simulink model "ASM_Traffic_V2X_Complete_Model_2"  (R2019a)
settings: Solver=ode1  StartTime=SIM.tstart.v  StopTime=Inf  FixedStep=SIM.StepSize.v  RelTol=1e-3
PostLoadFcn:
  | if any(exist('dsrtsu_mdlpostloadfcn', 'file') ~= 0), dsrtsu_mdlpostloadfcn('Execute', bdroot); end
  | try, asm_mdl_postloadfcn(bdroot, 'UpdateModel', 2200); catch, disp(lasterr); end,
undefined symbols (not defined in the file): _SensorPnts_1, _SensorPnts_13, _SensorPnts_17, _SensorPnts_21, _SensorPnts_25, _SensorPnts_29, _SensorPnts_33, _SensorPnts_37, _SensorPnts_41, _SensorPnts_45, _SensorPnts_49, _SensorPnts_5, _SensorPnts_53, _SensorPnts_57, _SensorPnts_9, _to_, CPT, G5A, ITS, MDL, rad, s_to_rpm, SIM
libraries: simulink x169, ASM_VehicleDynamics_lib x126, ASM_Traffic_lib x83, ASM_Utils_lib x49, mdbs x45, ASM_Environment_lib x17, dspindex x12, dsaV2xLibraryAux x10, dsmpblib x6, dsaV2xAsn1Library x4, dsaV2xLibrary x4, ASM_BrakeHydraulics_lib x4
(part 21 of 36)

== system ASM_Traffic_V2X_Complete_Model_2/MDLUserInterface/Environment/MDL_DISP/Traffic/Fellow_Movement ==
  TrafficBus : Inport
  CurrentSegment[] : Subsystem
      mask Display: disp('')
  CurrentSegment[]1 : Subsystem
      mask Display: disp('')
  CurrentSegment[]2 : Subsystem
      mask Display: disp('')
  CurrentSequence[] : Subsystem
      mask Display: disp('')
  CurrentSequence[]1 : Subsystem
      mask Display: disp('')
  CurrentSequence[]2 : Subsystem
      mask Display: disp('')
  Fellow_Movement_1 : Scope  NumInputPorts=7
  Fellow_Movement_2 : Scope  NumInputPorts=7
  Fellow_Movement_3 : Scope  NumInputPorts=7
  FlagFellowUsed[0|1] : Subsystem
      mask Display: disp('')
  FlagFellowUsed[0|1]1 : Subsystem
      mask Display: disp('')
  FlagFellowUsed[0|1]2 : Subsystem
      mask Display: disp('')
  GetFellowDataByIndex_1 : Subsystem
  GetFellowDataByIndex_2 : Subsystem
  GetFellowDataByIndex_3 : Subsystem
  SelectFellowDataByIndex_1 : Constant
  SelectFellowDataByIndex_2 : Constant  Value=2
  SelectFellowDataByIndex_3 : Constant  Value=3
  d_Total_Fellow[m] : Subsystem
      mask Display: disp('')
  d_Total_Fellow[m]1 : Subsystem
      mask Display: disp('')
  d_Total_Fellow[m]2 : Subsystem
      mask Display: disp('')
  s_Fellow[m] : Subsystem
      mask Display: disp('')
  s_Fellow[m]1 : Subsystem
      mask Display: disp('')
  s_Fellow[m]2 : Subsystem
      mask Display: disp('')
  t_local[s] : Subsystem
      mask Display: disp('')
  t_local[s]1 : Subsystem
      mask Display: disp('')
  t_local[s]2 : Subsystem
      mask Display: disp('')
  v_Fellow[km|h] : Subsystem
      mask Display: disp('')
  v_Fellow[km|h]1 : Subsystem
      mask Display: disp('')
  v_Fellow[km|h]2 : Subsystem
      mask Display: disp('')
  wires:
  TrafficBus/1 -> GetFellowDataByIndex_3/2(TrafficBus), GetFellowDataByIndex_2/2(TrafficBus), GetFellowDataByIndex_1/2(TrafficBus)
  SelectFellowDataByIndex_1/1 -> GetFellowDataByIndex_1/1(SelectFellowDataByIndex)
  CurrentSequence[]/1(Out1) -> Fellow_Movement_1/1  "CurrentSequence[]"
  CurrentSegment[]/1(Out1) -> Fellow_Movement_1/2  "CurrentSegment[]"
  t_local[s]/1(Out1) -> Fellow_Movement_1/3  "t_local[s]"
  FlagFellowUsed[0|1]/1(Out1) -> Fellow_Movement_1/4  "FlagFellowUsed[0|1]"
  s_Fellow[m]/1(Out1) -> Fellow_Movement_1/5  "s_Fellow[m]"
  d_Total_Fellow[m]/1(Out1) -> Fellow_Movement_1/6  "d_Total_Fellow[m]"
  v_Fellow[km|h]/1(Out1) -> Fellow_Movement_1/7  "v_Fellow[km|h]"
  GetFellowDataByIndex_1/1(CurrentSequence[]) -> CurrentSequence[]/1(In1)
  GetFellowDataByIndex_1/2(CurrentSegment[]) -> CurrentSegment[]/1(In1)
  GetFellowDataByIndex_1/3(t_local[s]) -> t_local[s]/1(In1)
  GetFellowDataByIndex_1/4(FlagFellowUsed[0|1]) -> FlagFellowUsed[0|1]/1(In1)
  GetFellowDataByIndex_1/5(s_Fellow[m]) -> s_Fellow[m]/1(In1)
  GetFellowDataByIndex_1/6(d_Total_Fellow[m]) -> d_Total_Fellow[m]/1(In1)
  GetFellowDataByIndex_1/7(v_Fellow[km|h]) -> v_Fellow[km|h]/1(In1)
  SelectFellowDataByIndex_2/1 -> GetFellowDataByIndex_2/1(SelectFellowDataByIndex)
  CurrentSequence[]1/1(Out1) -> Fellow_Movement_2/1  "CurrentSequence[]"
  CurrentSegment[]1/1(Out1) -> Fellow_Movement_2/2  "CurrentSegment[]"
  t_local[s]1/1(Out1) -> Fellow_Movement_2/3  "t_local[s]"
  FlagFellowUsed[0|1]1/1(Out1) -> Fellow_Movement_2/4  "FlagFellowUsed[0|1]"
  s_Fellow[m]1/1(Out1) -> Fellow_Movement_2/5  "s_Fellow[m]"
  d_Total_Fellow[m]1/1(Out1) -> Fellow_Movement_2/6  "d_Total_Fellow[m]"
  v_Fellow[km|h]1/1(Out1) -> Fellow_Movement_2/7  "v_Fellow[km|h]"
  GetFellowDataByIndex_2/1(CurrentSequence[]) -> CurrentSequence[]1/1(In1)
  GetFellowDataByIndex_2/2(CurrentSegment[]) -> CurrentSegment[]1/1(In1)
  GetFellowDataByIndex_2/3(t_local[s]) -> t_local[s]1/1(In1)
  GetFellowDataByIndex_2/4(FlagFellowUsed[0|1]) -> FlagFellowUsed[0|1]1/1(In1)
  GetFellowDataByIndex_2/5(s_Fellow[m]) -> s_Fellow[m]1/1(In1)
  GetFellowDataByIndex_2/6(d_Total_Fellow[m]) -> d_Total_Fellow[m]1/1(In1)
  GetFellowDataByIndex_2/7(v_Fellow[km|h]) -> v_Fellow[km|h]1/1(In1)
  SelectFellowDataByIndex_3/1 -> GetFellowDataByIndex_3/1(SelectFellowDataByIndex)
  CurrentSequence[]2/1(Out1) -> Fellow_Movement_3/1  "CurrentSequence[]"
  CurrentSegment[]2/1(Out1) -> Fellow_Movement_3/2  "CurrentSegment[]"
  t_local[s]2/1(Out1) -> Fellow_Movement_3/3  "t_local[s]"
  FlagFellowUsed[0|1]2/1(Out1) -> Fellow_Movement_3/4  "FlagFellowUsed[0|1]"
  s_Fellow[m]2/1(Out1) -> Fellow_Movement_3/5  "s_Fellow[m]"
  d_Total_Fellow[m]2/1(Out1) -> Fellow_Movement_3/6  "d_Total_Fellow[m]"
  v_Fellow[km|h]2/1(Out1) -> Fellow_Movement_3/7  "v_Fellow[km|h]"
  GetFellowDataByIndex_3/1(CurrentSequence[]) -> CurrentSequence[]2/1(In1)
  GetFellowDataByIndex_3/2(CurrentSegment[]) -> CurrentSegment[]2/1(In1)
  GetFellowDataByIndex_3/3(t_local[s]) -> t_local[s]2/1(In1)
  GetFellowDataByIndex_3/4(FlagFellowUsed[0|1]) -> FlagFellowUsed[0|1]2/1(In1)
  GetFellowDataByIndex_3/5(s_Fellow[m]) -> s_Fellow[m]2/1(In1)
  GetFellowDataByIndex_3/6(d_Total_Fellow[m]) -> d_Total_Fellow[m]2/1(In1)
  GetFellowDataByIndex_3/7(v_Fellow[km|h]) -> v_Fellow[km|h]2/1(In1)

== system ASM_Traffic_V2X_Complete_Model_2/MDLUserInterface/Environment/MDL_DISP/Traffic/Line_Sensor ==
  note: LineSensor-Output not
      | fed into SignalBus due
      | to large amount of signal data.
  TrafficBus : Inport
  Bus Selector : BusSelector  OutputSignals=Sensors.Line_Sensor.Line_Sensor_1.Info
  Bus Selector1 : BusSelector  OutputSignals=LineSensor_Data_Valid[0|1|2],Num_Pnts_Detected_Road_Lanes[],Num_Pnts_Detected_Road_Shape_Lines[],Num_Pnts_Detected_Road_Shape_ContObj[],Num_Pnts_Detected_Junction_Borders[],Num_Pnts_Detected_Junction_Shape_Lines[],Num_Pnts_Detected_Junction_Shape_ContObj[]
  Data_Valid[0|1|2] : Subsystem
      mask Display: disp('')
  Line_Sensor_Info : Scope  NumInputPorts=7
  Num_Pnts_Detected_Junction_Borders[] : Subsystem
      mask Display: disp('')
  Num_Pnts_Detected_Junction_Shape_ContObj[] : Subsystem
      mask Display: disp('')
  Num_Pnts_Detected_Junction_Shape_Lines[] : Subsystem
      mask Display: disp('')
  Num_Pnts_Detected_Road_Lanes[] : Subsystem
      mask Display: disp('')
  Num_Pnts_Detected_Road_Shape_ContObj[] : Subsystem
      mask Display: disp('')
  Num_Pnts_Detected_Road_Shape_Lines[] : Subsystem
      mask Display: disp('')
  wires:
  TrafficBus/1 -> Bus Selector/1
  Num_Pnts_Detected_Road_Shape_Lines[]/1(Out1) -> Line_Sensor_Info/3  "Num_Pnts_Detected_Road_Shape_Lines[]"
  Bus Selector1/3 -> Num_Pnts_Detected_Road_Shape_Lines[]/1(In1)  "<Num_Pnts_Detected_Road_Shape_Lines[]>"
  Num_Pnts_Detected_Road_Lanes[]/1(Out1) -> Line_Sensor_Info/2  "Num_Pnts_Detected_Road_Lanes[]"
  Data_Valid[0|1|2]/1(Out1) -> Line_Sensor_Info/1  "Data_Valid[0|1|2]"
  Bus Selector1/2 -> Num_Pnts_Detected_Road_Lanes[]/1(In1)  "<Num_Pnts_Detected_Road_Lanes[]>"
  Bus Selector1/1 -> Data_Valid[0|1|2]/1(In1)  "<LineSensor_Data_Valid[0|1|2]>"
  Bus Selector/1 -> Bus Selector1/1  "<Info>"
  Bus Selector1/4 -> Num_Pnts_Detected_Road_Shape_ContObj[]/1(In1)  "<Num_Pnts_Detected_Road_Shape_ContObj[]>"
  Num_Pnts_Detected_Road_Shape_ContObj[]/1(Out1) -> Line_Sensor_Info/4  "Num_Pnts_Detected_Road_Shape_ContObj[]"
  Bus Selector1/5 -> Num_Pnts_Detected_Junction_Borders[]/1(In1)  "<Num_Pnts_Detected_Junction_Borders[]>"
  Num_Pnts_Detected_Junction_Borders[]/1(Out1) -> Line_Sensor_Info/5  "Num_Pnts_Detected_Junction_Borders[]"
  Bus Selector1/7 -> Num_Pnts_Detected_Junction_Shape_ContObj[]/1(In1)  "<Num_Pnts_Detected_Junction_Shape_ContObj[]>"
  Bus Selector1/6 -> Num_Pnts_Detected_Junction_Shape_Lines[]/1(In1)  "<Num_Pnts_Detected_Junction_Shape_Lines[]>"
  Num_Pnts_Detected_Junction_Shape_Lines[]/1(Out1) -> Line_Sensor_Info/6  "Num_Pnts_Detected_Junction_Shape_Lines[]"
  Num_Pnts_Detected_Junction_Shape_ContObj[]/1(Out1) -> Line_Sensor_Info/7  "Num_Pnts_Detected_Junction_Shape_ContObj[]"

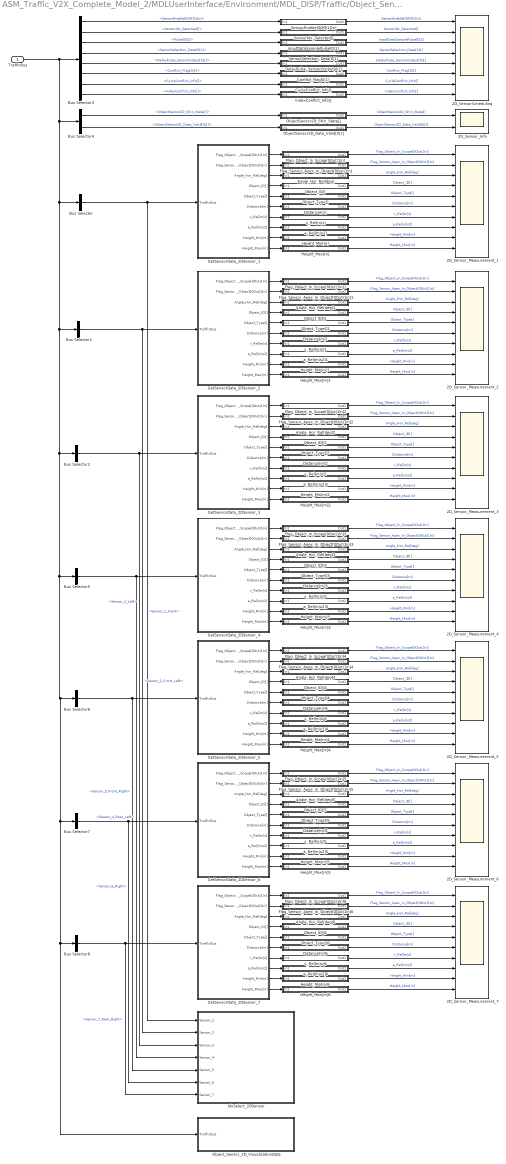
== system ASM_Traffic_V2X_Complete_Model_2/MDLUserInterface/Environment/MDL_DISP/Traffic/Object_Sensor_2D ==
  TrafficBus : Inport
  2D_SensorScheduling : Scope  NumInputPorts=8
  2D_Sensor_Info : Scope  NumInputPorts=2
  2D_Sensor_Measurement_{1..7} (7 alike) : Scope  NumInputPorts=10
  Angle_Hor_Rel[deg] : Subsystem
      mask Display: disp('')
  Angle_Hor_Rel[deg]1 : Subsystem
      mask Display: disp('')
  Angle_Hor_Rel[deg]2 : Subsystem
      mask Display: disp('')
  Angle_Hor_Rel[deg]3 : Subsystem
      mask Display: disp('')
  Angle_Hor_Rel[deg]4 : Subsystem
      mask Display: disp('')
  Angle_Hor_Rel[deg]5 : Subsystem
      mask Display: disp('')
  Angle_Hor_Rel[deg]6 : Subsystem
      mask Display: disp('')
  Bus Selector : BusSelector  OutputSignals=Sensors.Object_Sensor_2D.Sensor_1_Front
  Bus Selector1 : BusSelector  OutputSignals=Sensors.Object_Sensor_2D.Sensor_2_Front_Left
  Bus Selector2 : BusSelector  OutputSignals=Sensors.Object_Sensor_2D.Sensor_3_Left
  Bus Selector3 : BusSelector  OutputSignals=Sensors.Object_Sensor_2D.Sensor_Scheduler.SensorEnable[0Off|1On],Sensors.Object_Sensor_2D.Sensor_Scheduler.SensorIdx_Selected[],Sensors.Object_Sensor_2D.Sample_Pulse.Pulse[0|1],Sensors.Object_Sensor_2D.Sensor_Scheduler.SensorSelection_Data[0|1],Sensors.Object_Sensor_2D.Sensor_Scheduler.DelayPulse_SensorOutput[0|1],Sensors.Object_Sensor_2D.Sensor_Scheduler.Conflict_Flag[0|1],Sensors.Object_Sensor_2D.Sensor_Scheduler.CylceConflict_Info[],Sensors.Object_Sensor_2D.Sensor_Scheduler.IndexConflict_Info[]
  Bus Selector4 : BusSelector  OutputSignals=Sensors.Object_Sensor_2D.Sensor_1_Front.Info.ObjectSensor2D_Sfcn_State[],Sensors.Object_Sensor_2D.Sensor_1_Front.Info.ObjectSensor2D_Data_Valid[0|1]
  Bus Selector5 : BusSelector  OutputSignals=Sensors.Object_Sensor_2D.Sensor_4_Rear_Left
  Bus Selector6 : BusSelector  OutputSignals=Sensors.Object_Sensor_2D.Sensor_5_Front_Right
  Bus Selector7 : BusSelector  OutputSignals=Sensors.Object_Sensor_2D.Sensor_6_Right
  Bus Selector8 : BusSelector  OutputSignals=Sensors.Object_Sensor_2D.Sensor_7_Rear_Right
  Conflict_Flag[0|1] : Subsystem
      mask Display: disp('')
  CycleConflict_Info[] : Subsystem
      mask Display: disp('')
  DelayPulse_SensorOutput[0|1] : Subsystem
      mask Display: disp('')
  Distance[m] : Subsystem
      mask Display: disp('')
  Distance[m]1 : Subsystem
      mask Display: disp('')
  Distance[m]2 : Subsystem
      mask Display: disp('')
  Distance[m]3 : Subsystem
      mask Display: disp('')
  Distance[m]4 : Subsystem
      mask Display: disp('')
  Distance[m]5 : Subsystem
      mask Display: disp('')
  Distance[m]6 : Subsystem
      mask Display: disp('')
  Flag_Object_In_Scope[0Out|1In] : Subsystem
      mask Display: disp('')
  Flag_Object_In_Scope[0Out|1In]1 : Subsystem
      mask Display: disp('')
  Flag_Object_In_Scope[0Out|1In]2 : Subsystem
      mask Display: disp('')
  Flag_Object_In_Scope[0Out|1In]3 : Subsystem
      mask Display: disp('')
  Flag_Object_In_Scope[0Out|1In]4 : Subsystem
      mask Display: disp('')
  Flag_Object_In_Scope[0Out|1In]5 : Subsystem
      mask Display: disp('')
  Flag_Object_In_Scope[0Out|1In]6 : Subsystem
      mask Display: disp('')
  Flag_Sensor_Apex_In_Object[0Out|1In] : Subsystem
      mask Display: disp('')
  Flag_Sensor_Apex_In_Object[0Out|1In]1 : Subsystem
      mask Display: disp('')
  Flag_Sensor_Apex_In_Object[0Out|1In]2 : Subsystem
      mask Display: disp('')
  Flag_Sensor_Apex_In_Object[0Out|1In]3 : Subsystem
      mask Display: disp('')
  Flag_Sensor_Apex_In_Object[0Out|1In]4 : Subsystem
      mask Display: disp('')
  Flag_Sensor_Apex_In_Object[0Out|1In]5 : Subsystem
      mask Display: disp('')
  Flag_Sensor_Apex_In_Object[0Out|1In]6 : Subsystem
      mask Display: disp('')
  GetSensorData_2DSensor_1 : Subsystem
  GetSensorData_2DSensor_2 : Subsystem
  GetSensorData_2DSensor_3 : Subsystem
  GetSensorData_2DSensor_4 : Subsystem
  GetSensorData_2DSensor_5 : Subsystem
  GetSensorData_2DSensor_6 : Subsystem
  GetSensorData_2DSensor_7 : Subsystem
  Height_Max[m] : Subsystem
      mask Display: disp('')
  Height_Max[m]1 : Subsystem
      mask Display: disp('')
  Height_Max[m]2 : Subsystem
      mask Display: disp('')
  Height_Max[m]3 : Subsystem
      mask Display: disp('')
  Height_Max[m]4 : Subsystem
      mask Display: disp('')
  Height_Max[m]5 : Subsystem
      mask Display: disp('')
  Height_Max[m]6 : Subsystem
      mask Display: disp('')
  Height_Min[m] : Subsystem
      mask Display: disp('')
  Height_Min[m]1 : Subsystem
      mask Display: disp('')
  Height_Min[m]2 : Subsystem
      mask Display: disp('')
  Height_Min[m]3 : Subsystem
      mask Display: disp('')
  Height_Min[m]4 : Subsystem
      mask Display: disp('')
  Height_Min[m]5 : Subsystem
      mask Display: disp('')
  Height_Min[m]6 : Subsystem
      mask Display: disp('')
  IdxSelect_2DSensor : Subsystem
  IndexConflict_Info[] : Subsystem
      mask Display: disp('')
  InputDataSamplePulse[0|1] : Subsystem
      mask Display: disp('')
  ObjectSensor2D_Data_Valid[0|1] : Subsystem
      mask Display: disp('')
  ObjectSensor2D_Sfcn_State[] : Subsystem
      mask Display: disp('')
  Object_ID[] : Subsystem
      mask Display: disp('')
  Object_ID[]1 : Subsystem
      mask Display: disp('')
  Object_ID[]2 : Subsystem
      mask Display: disp('')
  Object_ID[]3 : Subsystem
      mask Display: disp('')
  Object_ID[]4 : Subsystem
      mask Display: disp('')
  Object_ID[]5 : Subsystem
      mask Display: disp('')
  Object_ID[]6 : Subsystem
      mask Display: disp('')
  Object_Sensor_2D_VisualizationData : Subsystem
  Object_Type[] : Subsystem
      mask Display: disp('')
  Object_Type[]1 : Subsystem
      mask Display: disp('')
  Object_Type[]2 : Subsystem
      mask Display: disp('')
  Object_Type[]3 : Subsystem
      mask Display: disp('')
  Object_Type[]4 : Subsystem
      mask Display: disp('')
  Object_Type[]5 : Subsystem
      mask Display: disp('')
  Object_Type[]6 : Subsystem
      mask Display: disp('')
  SensorEnable[0Off|1On] : Subsystem
      mask Display: disp('')
  SensorIdx_Selected[] : Subsystem
      mask Display: disp('')
  SensorSelection_Data[0|1] : Subsystem
      mask Display: disp('')
  a_Rel[m|s2] : Subsystem
      mask Display: disp('')
  a_Rel[m|s2]1 : Subsystem
      mask Display: disp('')
  a_Rel[m|s2]2 : Subsystem
      mask Display: disp('')
  a_Rel[m|s2]3 : Subsystem
      mask Display: disp('')
  a_Rel[m|s2]4 : Subsystem
      mask Display: disp('')
  a_Rel[m|s2]5 : Subsystem
      mask Display: disp('')
  a_Rel[m|s2]6 : Subsystem
      mask Display: disp('')
  v_Rel[m|s] : Subsystem
      mask Display: disp('')
  v_Rel[m|s]1 : Subsystem
      mask Display: disp('')
  v_Rel[m|s]2 : Subsystem
      mask Display: disp('')
  v_Rel[m|s]3 : Subsystem
      mask Display: disp('')
  v_Rel[m|s]4 : Subsystem
      mask Display: disp('')
  v_Rel[m|s]5 : Subsystem
      mask Display: disp('')
  v_Rel[m|s]6 : Subsystem
      mask Display: disp('')
  wires:
  GetSensorData_2DSensor_1/3(Angle_Hor_Rel[deg]) -> Angle_Hor_Rel[deg]/1(In1)
  GetSensorData_2DSensor_1/4(Object_ID[]) -> Object_ID[]/1(In1)
  GetSensorData_2DSensor_1/5(Object_Type[]) -> Object_Type[]/1(In1)
  GetSensorData_2DSensor_1/6(Distance[m]) -> Distance[m]/1(In1)
  GetSensorData_2DSensor_1/7(v_Rel[m|s]) -> v_Rel[m|s]/1(In1)
  GetSensorData_2DSensor_1/8(a_Rel[m|s2]) -> a_Rel[m|s2]/1(In1)
  GetSensorData_2DSensor_1/10(Height_Max[m]) -> Height_Max[m]/1(In1)
  GetSensorData_2DSensor_1/9(Height_Min[m]) -> Height_Min[m]/1(In1)
  Object_ID[]/1(Out1) -> 2D_Sensor_Measurement_1/4  "Object_ID[]"
  Object_Type[]/1(Out1) -> 2D_Sensor_Measurement_1/5  "Object_Type[]"
  Distance[m]/1(Out1) -> 2D_Sensor_Measurement_1/6  "Distance[m]"
  v_Rel[m|s]/1(Out1) -> 2D_Sensor_Measurement_1/7  "v_Rel[m|s]"
  a_Rel[m|s2]/1(Out1) -> 2D_Sensor_Measurement_1/8  "a_Rel[m|s2]"
  Height_Max[m]/1(Out1) -> 2D_Sensor_Measurement_1/10  "Height_Max[m]"
  Height_Min[m]/1(Out1) -> 2D_Sensor_Measurement_1/9  "Height_Min[m]"
  Bus Selector/1 -> GetSensorData_2DSensor_1/1(TrafficBus), IdxSelect_2DSensor/1(Sensor_1)  "<Sensor_1_Front>"
  Bus Selector3/4 -> SensorSelection_Data[0|1]/1(In1)  "<SensorSelection_Data[0|1]>"
  Bus Selector3/5 -> DelayPulse_SensorOutput[0|1]/1(In1)  "<DelayPulse_SensorOutput[0|1]>"
  Bus Selector3/6 -> Conflict_Flag[0|1]/1(In1)  "<Conflict_Flag[0|1]>"
  SensorEnable[0Off|1On]/1(Out1) -> 2D_SensorScheduling/1  "SensorEnable[0Off|1On]"
  InputDataSamplePulse[0|1]/1(Out1) -> 2D_SensorScheduling/3  "InputDataSamplePulse[0|1]"
  Bus Selector3/1 -> SensorEnable[0Off|1On]/1(In1)  "<SensorEnable[0Off|1On]>"
  Bus Selector3/3 -> InputDataSamplePulse[0|1]/1(In1)  "<Pulse[0|1]>"
  SensorSelection_Data[0|1]/1(Out1) -> 2D_SensorScheduling/4  "SensorSelection_Data[0|1]"
  DelayPulse_SensorOutput[0|1]/1(Out1) -> 2D_SensorScheduling/5  "DelayPulse_SensorOutput[0|1]"
  Conflict_Flag[0|1]/1(Out1) -> 2D_SensorScheduling/6  "Conflict_Flag[0|1]"
  CycleConflict_Info[]/1(Out1) -> 2D_SensorScheduling/7  "CycleConflict_Info[]"
  Bus Selector3/2 -> SensorIdx_Selected[]/1(In1)  "<SensorIdx_Selected[]>"
  Bus Selector3/7 -> CycleConflict_Info[]/1(In1)  "<CylceConflict_Info[]>"
  Bus Selector3/8 -> IndexConflict_Info[]/1(In1)  "<IndexConflict_Info[]>"
  IndexConflict_Info[]/1(Out1) -> 2D_SensorScheduling/8  "IndexConflict_Info[]"
  SensorIdx_Selected[]/1(Out1) -> 2D_SensorScheduling/2  "SensorIdx_Selected[]"
  Angle_Hor_Rel[deg]/1(Out1) -> 2D_Sensor_Measurement_1/3  "Angle_Hor_Rel[deg]"
  Bus Selector4/1 -> ObjectSensor2D_Sfcn_State[]/1(In1)  "<ObjectSensor2D_Sfcn_State[]>"
  Bus Selector4/2 -> ObjectSensor2D_Data_Valid[0|1]/1(In1)  "<ObjectSensor2D_Data_Valid[0|1]>"
  ObjectSensor2D_Sfcn_State[]/1(Out1) -> 2D_Sensor_Info/1  "ObjectSensor2D_Sfcn_State[]"
  ObjectSensor2D_Data_Valid[0|1]/1(Out1) -> 2D_Sensor_Info/2  "ObjectSensor2D_Data_Valid[0|1]"
  Bus Selector1/1 -> GetSensorData_2DSensor_2/1(TrafficBus), IdxSelect_2DSensor/2(Sensor_2)  "<Sensor_2_Front_Left>"
  Flag_Sensor_Apex_In_Object[0Out|1In]/1(Out1) -> 2D_Sensor_Measurement_1/2  "Flag_Sensor_Apex_In_Object[0Out|1In]"
  Flag_Object_In_Scope[0Out|1In]/1(Out1) -> 2D_Sensor_Measurement_1/1  "Flag_Object_In_Scope[0Out|1In]"
  GetSensorData_2DSensor_1/2(Flag_Sensor_Apex_In_Object[0Out|1In]) -> Flag_Sensor_Apex_In_Object[0Out|1In]/1(In1)
  GetSensorData_2DSensor_1/1(Flag_Object_In_Scope[0Out|1In]) -> Flag_Object_In_Scope[0Out|1In]/1(In1)
  GetSensorData_2DSensor_2/3(Angle_Hor_Rel[deg]) -> Angle_Hor_Rel[deg]1/1(In1)
  GetSensorData_2DSensor_2/4(Object_ID[]) -> Object_ID[]1/1(In1)
  GetSensorData_2DSensor_2/5(Object_Type[]) -> Object_Type[]1/1(In1)
  GetSensorData_2DSensor_2/6(Distance[m]) -> Distance[m]1/1(In1)
  GetSensorData_2DSensor_2/7(v_Rel[m|s]) -> v_Rel[m|s]1/1(In1)
  GetSensorData_2DSensor_2/8(a_Rel[m|s2]) -> a_Rel[m|s2]1/1(In1)
  GetSensorData_2DSensor_2/10(Height_Max[m]) -> Height_Max[m]1/1(In1)
  GetSensorData_2DSensor_2/9(Height_Min[m]) -> Height_Min[m]1/1(In1)
  Object_ID[]1/1(Out1) -> 2D_Sensor_Measurement_2/4  "Object_ID[]"
  Object_Type[]1/1(Out1) -> 2D_Sensor_Measurement_2/5  "Object_Type[]"
  Distance[m]1/1(Out1) -> 2D_Sensor_Measurement_2/6  "Distance[m]"
  v_Rel[m|s]1/1(Out1) -> 2D_Sensor_Measurement_2/7  "v_Rel[m|s]"
  a_Rel[m|s2]1/1(Out1) -> 2D_Sensor_Measurement_2/8  "a_Rel[m|s2]"
  Height_Max[m]1/1(Out1) -> 2D_Sensor_Measurement_2/10  "Height_Max[m]"
  Height_Min[m]1/1(Out1) -> 2D_Sensor_Measurement_2/9  "Height_Min[m]"
  Angle_Hor_Rel[deg]1/1(Out1) -> 2D_Sensor_Measurement_2/3  "Angle_Hor_Rel[deg]"
  Flag_Sensor_Apex_In_Object[0Out|1In]1/1(Out1) -> 2D_Sensor_Measurement_2/2  "Flag_Sensor_Apex_In_Object[0Out|1In]"
  Flag_Object_In_Scope[0Out|1In]1/1(Out1) -> 2D_Sensor_Measurement_2/1  "Flag_Object_In_Scope[0Out|1In]"
  GetSensorData_2DSensor_2/2(Flag_Sensor_Apex_In_Object[0Out|1In]) -> Flag_Sensor_Apex_In_Object[0Out|1In]1/1(In1)
  GetSensorData_2DSensor_2/1(Flag_Object_In_Scope[0Out|1In]) -> Flag_Object_In_Scope[0Out|1In]1/1(In1)
  Bus Selector2/1 -> GetSensorData_2DSensor_3/1(TrafficBus), IdxSelect_2DSensor/3(Sensor_3)  "<Sensor_3_Left>"
  GetSensorData_2DSensor_3/3(Angle_Hor_Rel[deg]) -> Angle_Hor_Rel[deg]2/1(In1)
  GetSensorData_2DSensor_3/4(Object_ID[]) -> Object_ID[]2/1(In1)
  GetSensorData_2DSensor_3/5(Object_Type[]) -> Object_Type[]2/1(In1)
  GetSensorData_2DSensor_3/6(Distance[m]) -> Distance[m]2/1(In1)
  GetSensorData_2DSensor_3/7(v_Rel[m|s]) -> v_Rel[m|s]2/1(In1)
  GetSensorData_2DSensor_3/8(a_Rel[m|s2]) -> a_Rel[m|s2]2/1(In1)
  GetSensorData_2DSensor_3/10(Height_Max[m]) -> Height_Max[m]2/1(In1)
  GetSensorData_2DSensor_3/9(Height_Min[m]) -> Height_Min[m]2/1(In1)
  Object_ID[]2/1(Out1) -> 2D_Sensor_Measurement_3/4  "Object_ID[]"
  Object_Type[]2/1(Out1) -> 2D_Sensor_Measurement_3/5  "Object_Type[]"
  Distance[m]2/1(Out1) -> 2D_Sensor_Measurement_3/6  "Distance[m]"
  v_Rel[m|s]2/1(Out1) -> 2D_Sensor_Measurement_3/7  "v_Rel[m|s]"
  a_Rel[m|s2]2/1(Out1) -> 2D_Sensor_Measurement_3/8  "a_Rel[m|s2]"
  Height_Max[m]2/1(Out1) -> 2D_Sensor_Measurement_3/10  "Height_Max[m]"
  Height_Min[m]2/1(Out1) -> 2D_Sensor_Measurement_3/9  "Height_Min[m]"
  Angle_Hor_Rel[deg]2/1(Out1) -> 2D_Sensor_Measurement_3/3  "Angle_Hor_Rel[deg]"
  Flag_Sensor_Apex_In_Object[0Out|1In]2/1(Out1) -> 2D_Sensor_Measurement_3/2  "Flag_Sensor_Apex_In_Object[0Out|1In]"
  Flag_Object_In_Scope[0Out|1In]2/1(Out1) -> 2D_Sensor_Measurement_3/1  "Flag_Object_In_Scope[0Out|1In]"
  GetSensorData_2DSensor_3/2(Flag_Sensor_Apex_In_Object[0Out|1In]) -> Flag_Sensor_Apex_In_Object[0Out|1In]2/1(In1)
  GetSensorData_2DSensor_3/1(Flag_Object_In_Scope[0Out|1In]) -> Flag_Object_In_Scope[0Out|1In]2/1(In1)
  Bus Selector5/1 -> GetSensorData_2DSensor_4/1(TrafficBus), IdxSelect_2DSensor/4(Sensor_4)  "<Sensor_4_Rear_Left>"
  GetSensorData_2DSensor_4/3(Angle_Hor_Rel[deg]) -> Angle_Hor_Rel[deg]3/1(In1)
  GetSensorData_2DSensor_4/4(Object_ID[]) -> Object_ID[]3/1(In1)
  GetSensorData_2DSensor_4/5(Object_Type[]) -> Object_Type[]3/1(In1)
  GetSensorData_2DSensor_4/6(Distance[m]) -> Distance[m]3/1(In1)
  GetSensorData_2DSensor_4/7(v_Rel[m|s]) -> v_Rel[m|s]3/1(In1)
  GetSensorData_2DSensor_4/8(a_Rel[m|s2]) -> a_Rel[m|s2]3/1(In1)
  GetSensorData_2DSensor_4/10(Height_Max[m]) -> Height_Max[m]3/1(In1)
  GetSensorData_2DSensor_4/9(Height_Min[m]) -> Height_Min[m]3/1(In1)
  Object_ID[]3/1(Out1) -> 2D_Sensor_Measurement_4/4  "Object_ID[]"
  Object_Type[]3/1(Out1) -> 2D_Sensor_Measurement_4/5  "Object_Type[]"
  Distance[m]3/1(Out1) -> 2D_Sensor_Measurement_4/6  "Distance[m]"
  v_Rel[m|s]3/1(Out1) -> 2D_Sensor_Measurement_4/7  "v_Rel[m|s]"
  a_Rel[m|s2]3/1(Out1) -> 2D_Sensor_Measurement_4/8  "a_Rel[m|s2]"
  Height_Max[m]3/1(Out1) -> 2D_Sensor_Measurement_4/10  "Height_Max[m]"
  Height_Min[m]3/1(Out1) -> 2D_Sensor_Measurement_4/9  "Height_Min[m]"
  Angle_Hor_Rel[deg]3/1(Out1) -> 2D_Sensor_Measurement_4/3  "Angle_Hor_Rel[deg]"
  Flag_Sensor_Apex_In_Object[0Out|1In]3/1(Out1) -> 2D_Sensor_Measurement_4/2  "Flag_Sensor_Apex_In_Object[0Out|1In]"
  Flag_Object_In_Scope[0Out|1In]3/1(Out1) -> 2D_Sensor_Measurement_4/1  "Flag_Object_In_Scope[0Out|1In]"
  GetSensorData_2DSensor_4/2(Flag_Sensor_Apex_In_Object[0Out|1In]) -> Flag_Sensor_Apex_In_Object[0Out|1In]3/1(In1)
  GetSensorData_2DSensor_4/1(Flag_Object_In_Scope[0Out|1In]) -> Flag_Object_In_Scope[0Out|1In]3/1(In1)
  Bus Selector6/1 -> GetSensorData_2DSensor_5/1(TrafficBus), IdxSelect_2DSensor/5(Sensor_5)  "<Sensor_5_Front_Right>"
  GetSensorData_2DSensor_5/3(Angle_Hor_Rel[deg]) -> Angle_Hor_Rel[deg]4/1(In1)
  GetSensorData_2DSensor_5/4(Object_ID[]) -> Object_ID[]4/1(In1)
  GetSensorData_2DSensor_5/5(Object_Type[]) -> Object_Type[]4/1(In1)
  GetSensorData_2DSensor_5/6(Distance[m]) -> Distance[m]4/1(In1)
  GetSensorData_2DSensor_5/7(v_Rel[m|s]) -> v_Rel[m|s]4/1(In1)
  GetSensorData_2DSensor_5/8(a_Rel[m|s2]) -> a_Rel[m|s2]4/1(In1)
  GetSensorData_2DSensor_5/10(Height_Max[m]) -> Height_Max[m]4/1(In1)
  GetSensorData_2DSensor_5/9(Height_Min[m]) -> Height_Min[m]4/1(In1)
  Object_ID[]4/1(Out1) -> 2D_Sensor_Measurement_5/4  "Object_ID[]"
  Object_Type[]4/1(Out1) -> 2D_Sensor_Measurement_5/5  "Object_Type[]"
  Distance[m]4/1(Out1) -> 2D_Sensor_Measurement_5/6  "Distance[m]"
  v_Rel[m|s]4/1(Out1) -> 2D_Sensor_Measurement_5/7  "v_Rel[m|s]"
  a_Rel[m|s2]4/1(Out1) -> 2D_Sensor_Measurement_5/8  "a_Rel[m|s2]"
  Height_Max[m]4/1(Out1) -> 2D_Sensor_Measurement_5/10  "Height_Max[m]"
  Height_Min[m]4/1(Out1) -> 2D_Sensor_Measurement_5/9  "Height_Min[m]"
  Angle_Hor_Rel[deg]4/1(Out1) -> 2D_Sensor_Measurement_5/3  "Angle_Hor_Rel[deg]"
  Flag_Sensor_Apex_In_Object[0Out|1In]4/1(Out1) -> 2D_Sensor_Measurement_5/2  "Flag_Sensor_Apex_In_Object[0Out|1In]"
  Flag_Object_In_Scope[0Out|1In]4/1(Out1) -> 2D_Sensor_Measurement_5/1  "Flag_Object_In_Scope[0Out|1In]"
  GetSensorData_2DSensor_5/2(Flag_Sensor_Apex_In_Object[0Out|1In]) -> Flag_Sensor_Apex_In_Object[0Out|1In]4/1(In1)
  GetSensorData_2DSensor_5/1(Flag_Object_In_Scope[0Out|1In]) -> Flag_Object_In_Scope[0Out|1In]4/1(In1)
  Bus Selector7/1 -> GetSensorData_2DSensor_6/1(TrafficBus), IdxSelect_2DSensor/6(Sensor_6)  "<Sensor_6_Right>"
  GetSensorData_2DSensor_6/3(Angle_Hor_Rel[deg]) -> Angle_Hor_Rel[deg]5/1(In1)
  GetSensorData_2DSensor_6/4(Object_ID[]) -> Object_ID[]5/1(In1)
  GetSensorData_2DSensor_6/5(Object_Type[]) -> Object_Type[]5/1(In1)
  GetSensorData_2DSensor_6/6(Distance[m]) -> Distance[m]5/1(In1)
  GetSensorData_2DSensor_6/7(v_Rel[m|s]) -> v_Rel[m|s]5/1(In1)
  GetSensorData_2DSensor_6/8(a_Rel[m|s2]) -> a_Rel[m|s2]5/1(In1)
  GetSensorData_2DSensor_6/10(Height_Max[m]) -> Height_Max[m]5/1(In1)
  GetSensorData_2DSensor_6/9(Height_Min[m]) -> Height_Min[m]5/1(In1)
  Object_ID[]5/1(Out1) -> 2D_Sensor_Measurement_6/4  "Object_ID[]"
  Object_Type[]5/1(Out1) -> 2D_Sensor_Measurement_6/5  "Object_Type[]"
  Distance[m]5/1(Out1) -> 2D_Sensor_Measurement_6/6  "Distance[m]"
  v_Rel[m|s]5/1(Out1) -> 2D_Sensor_Measurement_6/7  "v_Rel[m|s]"
  a_Rel[m|s2]5/1(Out1) -> 2D_Sensor_Measurement_6/8  "a_Rel[m|s2]"
  Height_Max[m]5/1(Out1) -> 2D_Sensor_Measurement_6/10  "Height_Max[m]"
  Height_Min[m]5/1(Out1) -> 2D_Sensor_Measurement_6/9  "Height_Min[m]"
  Angle_Hor_Rel[deg]5/1(Out1) -> 2D_Sensor_Measurement_6/3  "Angle_Hor_Rel[deg]"
  Flag_Sensor_Apex_In_Object[0Out|1In]5/1(Out1) -> 2D_Sensor_Measurement_6/2  "Flag_Sensor_Apex_In_Object[0Out|1In]"
  Flag_Object_In_Scope[0Out|1In]5/1(Out1) -> 2D_Sensor_Measurement_6/1  "Flag_Object_In_Scope[0Out|1In]"
  GetSensorData_2DSensor_6/2(Flag_Sensor_Apex_In_Object[0Out|1In]) -> Flag_Sensor_Apex_In_Object[0Out|1In]5/1(In1)
  GetSensorData_2DSensor_6/1(Flag_Object_In_Scope[0Out|1In]) -> Flag_Object_In_Scope[0Out|1In]5/1(In1)
  TrafficBus/1 -> Object_Sensor_2D_VisualizationData/1(TrafficBus), Bus Selector8/1, Bus Selector7/1, Bus Selector6/1, Bus Selector5/1, Bus Selector2/1, Bus Selector1/1, Bus Selector/1, Bus Selector4/1, Bus Selector3/1
  Bus Selector8/1 -> IdxSelect_2DSensor/7(Sensor_7), GetSensorData_2DSensor_7/1(TrafficBus)  "<Sensor_7_Rear_Right>"
  GetSensorData_2DSensor_7/3(Angle_Hor_Rel[deg]) -> Angle_Hor_Rel[deg]6/1(In1)
  GetSensorData_2DSensor_7/4(Object_ID[]) -> Object_ID[]6/1(In1)
  GetSensorData_2DSensor_7/5(Object_Type[]) -> Object_Type[]6/1(In1)
  GetSensorData_2DSensor_7/6(Distance[m]) -> Distance[m]6/1(In1)
  GetSensorData_2DSensor_7/7(v_Rel[m|s]) -> v_Rel[m|s]6/1(In1)
  GetSensorData_2DSensor_7/8(a_Rel[m|s2]) -> a_Rel[m|s2]6/1(In1)
  GetSensorData_2DSensor_7/10(Height_Max[m]) -> Height_Max[m]6/1(In1)
  GetSensorData_2DSensor_7/9(Height_Min[m]) -> Height_Min[m]6/1(In1)
  Object_ID[]6/1(Out1) -> 2D_Sensor_Measurement_7/4  "Object_ID[]"
  Object_Type[]6/1(Out1) -> 2D_Sensor_Measurement_7/5  "Object_Type[]"
  Distance[m]6/1(Out1) -> 2D_Sensor_Measurement_7/6  "Distance[m]"
  v_Rel[m|s]6/1(Out1) -> 2D_Sensor_Measurement_7/7  "v_Rel[m|s]"
  a_Rel[m|s2]6/1(Out1) -> 2D_Sensor_Measurement_7/8  "a_Rel[m|s2]"
  Height_Max[m]6/1(Out1) -> 2D_Sensor_Measurement_7/10  "Height_Max[m]"
  Height_Min[m]6/1(Out1) -> 2D_Sensor_Measurement_7/9  "Height_Min[m]"
  Angle_Hor_Rel[deg]6/1(Out1) -> 2D_Sensor_Measurement_7/3  "Angle_Hor_Rel[deg]"
  Flag_Sensor_Apex_In_Object[0Out|1In]6/1(Out1) -> 2D_Sensor_Measurement_7/2  "Flag_Sensor_Apex_In_Object[0Out|1In]"
  Flag_Object_In_Scope[0Out|1In]6/1(Out1) -> 2D_Sensor_Measurement_7/1  "Flag_Object_In_Scope[0Out|1In]"
  GetSensorData_2DSensor_7/2(Flag_Sensor_Apex_In_Object[0Out|1In]) -> Flag_Sensor_Apex_In_Object[0Out|1In]6/1(In1)
  GetSensorData_2DSensor_7/1(Flag_Object_In_Scope[0Out|1In]) -> Flag_Object_In_Scope[0Out|1In]6/1(In1)

== system ASM_Traffic_V2X_Complete_Model_2/MDLUserInterface/Environment/MDL_DISP/Traffic/Object_Sensor_3D ==
  TrafficBus : Inport
  3D_Sensor_Info_1 : Scope  NumInputPorts=5
  3D_Sensor_Info_2 : Scope  NumInputPorts=5
  3D_Sensor_Info_3 : Scope  NumInputPorts=5
  3D_Sensor_Measurement_1 : Scope  NumInputPorts=7
  3D_Sensor_Measurement_2 : Scope  NumInputPorts=7
  3D_Sensor_Measurement_3 : Scope  NumInputPorts=7
  Angle_Hor_Object[deg] : Subsystem
      mask Display: disp('')
  Angle_Hor_Object[deg]1 : Subsystem
      mask Display: disp('')
  Angle_Hor_Object[deg]2 : Subsystem
      mask Display: disp('')
  Angle_Ver_Object[deg] : Subsystem
      mask Display: disp('')
  Angle_Ver_Object[deg]1 : Subsystem
      mask Display: disp('')
  Angle_Ver_Object[deg]2 : Subsystem
      mask Display: disp('')
  Bus Selector : BusSelector  OutputSignals=Sensors.Object_Sensor_3D.Sensor_1_Front_Long
  Bus Selector1 : BusSelector  OutputSignals=Sensors.Object_Sensor_3D.Sensor_2_Front_Mid
  Bus Selector2 : BusSelector  OutputSignals=Sensors.Object_Sensor_3D.Sensor_3_Rear
  Bus Selector3 : BusSelector  OutputSignals=Sensors.Object_Sensor_3D.Sensor_Scheduler.SensorEnable[0Off|1On],Sensors.Object_Sensor_3D.Sensor_Scheduler.SensorIdx_Selected[],Sensors.Object_Sensor_3D.Sample_Pulse.Pulse[0|1],Sensors.Object_Sensor_3D.Sensor_Scheduler.SensorSelection_Data[0|1],Sensors.Object_Sensor_3D.Sensor_Scheduler.DelayPulse_SensorOutput[0|1],Sensors.Object_Sensor_3D.Sensor_Scheduler.Conflict_Flag[0|1],Sensors.Object_Sensor_3D.Sensor_Scheduler.CylceConflict_Info[],Sensors.Object_Sensor_3D.Sensor_Scheduler.IndexConflict_Info[]
  Conflict_Flag[0|1] : Subsystem
      mask Display: disp('')
  CycleConflict_Info[] : Subsystem
      mask Display: disp('')
  DelayPulse_SensorOutput[0|1] : Subsystem
      mask Display: disp('')
  Dist_Object[m] : Subsystem
      mask Display: disp('')
  Dist_Object[m]1 : Subsystem
      mask Display: disp('')
  Dist_Object[m]2 : Subsystem
      mask Display: disp('')
  Flag_NearestPnt_Occluded[-1|0|1] : Subsystem
      mask Display: disp('')
  Flag_NearestPnt_Occluded[-1|0|1]1 : Subsystem
      mask Display: disp('')
  Flag_NearestPnt_Occluded[-1|0|1]2 : Subsystem
      mask Display: disp('')
  Flag_Object_In_Scope[0Out|1In] : Subsystem
      mask Display: disp('')
  Flag_Object_In_Scope[0Out|1In]1 : Subsystem
      mask Display: disp('')
  Flag_Object_In_Scope[0Out|1In]2 : Subsystem
      mask Display: disp('')
  Flag_Sensor_Apex_In_Object[0Out|1In] : Subsystem
      mask Display: disp('')
  Flag_Sensor_Apex_In_Object[0Out|1In]1 : Subsystem
      mask Display: disp('')
  Flag_Sensor_Apex_In_Object[0Out|1In]2 : Subsystem
      mask Display: disp('')
  GetSensorData_3DSensor_1 : Subsystem
  GetSensorData_3DSensor_2 : Subsystem
  GetSensorData_3DSensor_3 : Subsystem
  IdxSelect_3DSensor : Subsystem
  IndexConflict_Info[] : Subsystem
      mask Display: disp('')
  InputDataSamplePulse[0|1] : Subsystem
      mask Display: disp('')
  Object_ID[] : Subsystem
      mask Display: disp('')
  Object_ID[]1 : Subsystem
      mask Display: disp('')
  Object_ID[]2 : Subsystem
      mask Display: disp('')
  Object_Info[-1None|1Fellow|2Static] : Subsystem
      mask Display: disp('')
  Object_Info[-1None|1Fellow|2Static]1 : Subsystem
      mask Display: disp('')
  Object_Info[-1None|1Fellow|2Static]2 : Subsystem
      mask Display: disp('')
  Object_Sensor_3D_VisualizationData : Subsystem
  Object_Type[] : Subsystem
      mask Display: disp('')
  Object_Type[]1 : Subsystem
      mask Display: disp('')
  Object_Type[]2 : Subsystem
      mask Display: disp('')
  Occlusion_Ratio_Object[-1|0_1] : Subsystem
      mask Display: disp('')
  Occlusion_Ratio_Object[-1|0_1]1 : Subsystem
      mask Display: disp('')
  Occlusion_Ratio_Object[-1|0_1]2 : Subsystem
      mask Display: disp('')
  SensorEnable[0Off|1On] : Subsystem
      mask Display: disp('')
  SensorIdx_Selected[] : Subsystem
      mask Display: disp('')
  SensorScheduling : Scope  NumInputPorts=8
  SensorSelection_Data[0|1] : Subsystem
      mask Display: disp('')
  a_Rel_Object[m|s2] : Subsystem
      mask Display: disp('')
  a_Rel_Object[m|s2]1 : Subsystem
      mask Display: disp('')
  a_Rel_Object[m|s2]2 : Subsystem
      mask Display: disp('')
  v_Rel_Object[m|s] : Subsystem
      mask Display: disp('')
  v_Rel_Object[m|s]1 : Subsystem
      mask Display: disp('')
  v_Rel_Object[m|s]2 : Subsystem
      mask Display: disp('')
  wires:
  SensorIdx_Selected[]/1(Out1) -> SensorScheduling/2  "SensorIdx_Selected[]"
  IndexConflict_Info[]/1(Out1) -> SensorScheduling/8  "IndexConflict_Info[]"
  Bus Selector3/8 -> IndexConflict_Info[]/1(In1)  "<IndexConflict_Info[]>"
  Bus Selector3/7 -> CycleConflict_Info[]/1(In1)  "<CylceConflict_Info[]>"
  Bus Selector3/2 -> SensorIdx_Selected[]/1(In1)  "<SensorIdx_Selected[]>"
  CycleConflict_Info[]/1(Out1) -> SensorScheduling/7  "CycleConflict_Info[]"
  Conflict_Flag[0|1]/1(Out1) -> SensorScheduling/6  "Conflict_Flag[0|1]"
  DelayPulse_SensorOutput[0|1]/1(Out1) -> SensorScheduling/5  "DelayPulse_SensorOutput[0|1]"
  SensorSelection_Data[0|1]/1(Out1) -> SensorScheduling/4  "SensorSelection_Data[0|1]"
  Bus Selector3/3 -> InputDataSamplePulse[0|1]/1(In1)  "<Pulse[0|1]>"
  Bus Selector3/1 -> SensorEnable[0Off|1On]/1(In1)  "<SensorEnable[0Off|1On]>"
  InputDataSamplePulse[0|1]/1(Out1) -> SensorScheduling/3  "InputDataSamplePulse[0|1]"
  SensorEnable[0Off|1On]/1(Out1) -> SensorScheduling/1  "SensorEnable[0Off|1On]"
  Bus Selector3/6 -> Conflict_Flag[0|1]/1(In1)  "<Conflict_Flag[0|1]>"
  Bus Selector3/5 -> DelayPulse_SensorOutput[0|1]/1(In1)  "<DelayPulse_SensorOutput[0|1]>"
  Bus Selector3/4 -> SensorSelection_Data[0|1]/1(In1)  "<SensorSelection_Data[0|1]>"
  Bus Selector2/1 -> IdxSelect_3DSensor/3(Sensor_3), GetSensorData_3DSensor_3/1(TrafficBus)  "<Sensor_3_Rear>"
  Bus Selector1/1 -> GetSensorData_3DSensor_2/1(TrafficBus), IdxSelect_3DSensor/2(Sensor_2)  "<Sensor_2_Front_Mid>"
  Bus Selector/1 -> GetSensorData_3DSensor_1/1(TrafficBus), IdxSelect_3DSensor/1(Sensor_1)  "<Sensor_1_Front_Long>"
  GetSensorData_3DSensor_3/10(Angle_Ver_Object[deg]) -> Angle_Ver_Object[deg]2/1(In1)
  GetSensorData_3DSensor_3/9(Angle_Hor_Object[deg]) -> Angle_Hor_Object[deg]2/1(In1)
  GetSensorData_3DSensor_3/8(a_Rel_Object[m|s2]) -> a_Rel_Object[m|s2]2/1(In1)
  GetSensorData_3DSensor_3/7(v_Rel_Object[m|s]) -> v_Rel_Object[m|s]2/1(In1)
  GetSensorData_3DSensor_3/6(Dist_Object[m]) -> Dist_Object[m]2/1(In1)
  GetSensorData_3DSensor_3/5(Object_Type[]) -> Object_Type[]2/1(In1)
  GetSensorData_3DSensor_3/4(Object_ID[]) -> Object_ID[]2/1(In1)
  GetSensorData_3DSensor_3/3(Object_Info[-1None|1Fellow|2Static]) -> Object_Info[-1None|1Fellow|2Static]2/1(In1)
  GetSensorData_3DSensor_3/2(Flag_Sensor_Apex_In_Object[0Out|1In]) -> Flag_Sensor_Apex_In_Object[0Out|1In]2/1(In1)
  GetSensorData_3DSensor_3/1(Flag_Object_In_Scope[0Out|1In]) -> Flag_Object_In_Scope[0Out|1In]2/1(In1)
  Angle_Ver_Object[deg]2/1(Out1) -> 3D_Sensor_Measurement_3/5  "Angle_Ver_Object[deg]"
  Angle_Hor_Object[deg]2/1(Out1) -> 3D_Sensor_Measurement_3/4  "Angle_Hor_Object[deg]"
  a_Rel_Object[m|s2]2/1(Out1) -> 3D_Sensor_Measurement_3/3  "a_Rel_Object[m|s2]"
  v_Rel_Object[m|s]2/1(Out1) -> 3D_Sensor_Measurement_3/2  "v_Rel_Object[m|s]"
  Dist_Object[m]2/1(Out1) -> 3D_Sensor_Measurement_3/1  "Dist_Object[m]"
  Object_Type[]2/1(Out1) -> 3D_Sensor_Info_3/5  "Object_Type[]"
  Object_ID[]2/1(Out1) -> 3D_Sensor_Info_3/4  "Object_ID[]"
  Object_Info[-1None|1Fellow|2Static]2/1(Out1) -> 3D_Sensor_Info_3/3  "Object_Info[-1None|1Fellow|2Static]"
  Flag_Sensor_Apex_In_Object[0Out|1In]2/1(Out1) -> 3D_Sensor_Info_3/2  "Flag_Sensor_Apex_In_Object[0Out|1In]"
  Flag_Object_In_Scope[0Out|1In]2/1(Out1) -> 3D_Sensor_Info_3/1  "Flag_Object_In_Scope[0Out|1In]"
  Angle_Ver_Object[deg]1/1(Out1) -> 3D_Sensor_Measurement_2/5  "Angle_Ver_Object[deg]"
  Angle_Hor_Object[deg]1/1(Out1) -> 3D_Sensor_Measurement_2/4  "Angle_Hor_Object[deg]"
  a_Rel_Object[m|s2]1/1(Out1) -> 3D_Sensor_Measurement_2/3  "a_Rel_Object[m|s2]"
  v_Rel_Object[m|s]1/1(Out1) -> 3D_Sensor_Measurement_2/2  "v_Rel_Object[m|s]"
  Dist_Object[m]1/1(Out1) -> 3D_Sensor_Measurement_2/1  "Dist_Object[m]"
  Object_Type[]1/1(Out1) -> 3D_Sensor_Info_2/5  "Object_Type[]"
  Object_ID[]1/1(Out1) -> 3D_Sensor_Info_2/4  "Object_ID[]"
  Object_Info[-1None|1Fellow|2Static]1/1(Out1) -> 3D_Sensor_Info_2/3  "Object_Info[-1None|1Fellow|2Static]"
  Flag_Sensor_Apex_In_Object[0Out|1In]1/1(Out1) -> 3D_Sensor_Info_2/2  "Flag_Sensor_Apex_In_Object[0Out|1In]"
  Flag_Object_In_Scope[0Out|1In]1/1(Out1) -> 3D_Sensor_Info_2/1  "Flag_Object_In_Scope[0Out|1In]"
  Angle_Ver_Object[deg]/1(Out1) -> 3D_Sensor_Measurement_1/5  "Angle_Ver_Object[deg]"
  Angle_Hor_Object[deg]/1(Out1) -> 3D_Sensor_Measurement_1/4  "Angle_Hor_Object[deg]"
  a_Rel_Object[m|s2]/1(Out1) -> 3D_Sensor_Measurement_1/3  "a_Rel_Object[m|s2]"
  v_Rel_Object[m|s]/1(Out1) -> 3D_Sensor_Measurement_1/2  "v_Rel_Object[m|s]"
  Dist_Object[m]/1(Out1) -> 3D_Sensor_Measurement_1/1  "Dist_Object[m]"
  Object_Type[]/1(Out1) -> 3D_Sensor_Info_1/5  "Object_Type[]"
  Object_ID[]/1(Out1) -> 3D_Sensor_Info_1/4  "Object_ID[]"
  Object_Info[-1None|1Fellow|2Static]/1(Out1) -> 3D_Sensor_Info_1/3  "Object_Info[-1None|1Fellow|2Static]"
  Flag_Sensor_Apex_In_Object[0Out|1In]/1(Out1) -> 3D_Sensor_Info_1/2  "Flag_Sensor_Apex_In_Object[0Out|1In]"
  Flag_Object_In_Scope[0Out|1In]/1(Out1) -> 3D_Sensor_Info_1/1  "Flag_Object_In_Scope[0Out|1In]"
  GetSensorData_3DSensor_1/10(Angle_Ver_Object[deg]) -> Angle_Ver_Object[deg]/1(In1)
  GetSensorData_3DSensor_1/9(Angle_Hor_Object[deg]) -> Angle_Hor_Object[deg]/1(In1)
  GetSensorData_3DSensor_1/8(a_Rel_Object[m|s2]) -> a_Rel_Object[m|s2]/1(In1)
  GetSensorData_3DSensor_1/7(v_Rel_Object[m|s]) -> v_Rel_Object[m|s]/1(In1)
  GetSensorData_3DSensor_1/6(Dist_Object[m]) -> Dist_Object[m]/1(In1)
  GetSensorData_3DSensor_1/5(Object_Type[]) -> Object_Type[]/1(In1)
  GetSensorData_3DSensor_1/4(Object_ID[]) -> Object_ID[]/1(In1)
  GetSensorData_3DSensor_1/3(Object_Info[-1None|1Fellow|2Static]) -> Object_Info[-1None|1Fellow|2Static]/1(In1)
  GetSensorData_3DSensor_1/2(Flag_Sensor_Apex_In_Object[0Out|1In]) -> Flag_Sensor_Apex_In_Object[0Out|1In]/1(In1)
  GetSensorData_3DSensor_1/1(Flag_Object_In_Scope[0Out|1In]) -> Flag_Object_In_Scope[0Out|1In]/1(In1)
  TrafficBus/1 -> Bus Selector3/1, Bus Selector/1, Object_Sensor_3D_VisualizationData/1(TrafficBus), Bus Selector2/1, Bus Selector1/1
  GetSensorData_3DSensor_1/11(Occlusion_Ratio_Object[-1|0_1]) -> Occlusion_Ratio_Object[-1|0_1]/1(In1)
  GetSensorData_3DSensor_1/12(Flag_NearestPnt_Occluded[-1|0|1]) -> Flag_NearestPnt_Occluded[-1|0|1]/1(In1)
  Occlusion_Ratio_Object[-1|0_1]/1(Out1) -> 3D_Sensor_Measurement_1/6  "Occlusion_Ratio_Object[-1|0_1]"
  Flag_NearestPnt_Occluded[-1|0|1]/1(Out1) -> 3D_Sensor_Measurement_1/7  "Flag_NearestPnt_Occluded[-1|0|1]"
  GetSensorData_3DSensor_2/1(Flag_Object_In_Scope[0Out|1In]) -> Flag_Object_In_Scope[0Out|1In]1/1(In1)
  GetSensorData_3DSensor_2/2(Flag_Sensor_Apex_In_Object[0Out|1In]) -> Flag_Sensor_Apex_In_Object[0Out|1In]1/1(In1)
  GetSensorData_3DSensor_2/3(Object_Info[-1None|1Fellow|2Static]) -> Object_Info[-1None|1Fellow|2Static]1/1(In1)
  GetSensorData_3DSensor_2/4(Object_ID[]) -> Object_ID[]1/1(In1)
  GetSensorData_3DSensor_2/5(Object_Type[]) -> Object_Type[]1/1(In1)
  GetSensorData_3DSensor_2/6(Dist_Object[m]) -> Dist_Object[m]1/1(In1)
  GetSensorData_3DSensor_2/7(v_Rel_Object[m|s]) -> v_Rel_Object[m|s]1/1(In1)
  GetSensorData_3DSensor_2/8(a_Rel_Object[m|s2]) -> a_Rel_Object[m|s2]1/1(In1)
  GetSensorData_3DSensor_2/9(Angle_Hor_Object[deg]) -> Angle_Hor_Object[deg]1/1(In1)
  GetSensorData_3DSensor_2/10(Angle_Ver_Object[deg]) -> Angle_Ver_Object[deg]1/1(In1)
  Flag_NearestPnt_Occluded[-1|0|1]1/1(Out1) -> 3D_Sensor_Measurement_2/7  "Flag_NearestPnt_Occluded[-1|0|1]"
  GetSensorData_3DSensor_2/12(Flag_NearestPnt_Occluded[-1|0|1]) -> Flag_NearestPnt_Occluded[-1|0|1]1/1(In1)
  Occlusion_Ratio_Object[-1|0_1]1/1(Out1) -> 3D_Sensor_Measurement_2/6  "Occlusion_Ratio_Object[-1|0_1]"
  GetSensorData_3DSensor_2/11(Occlusion_Ratio_Object[-1|0_1]) -> Occlusion_Ratio_Object[-1|0_1]1/1(In1)
  GetSensorData_3DSensor_3/11(Occlusion_Ratio_Object[-1|0_1]) -> Occlusion_Ratio_Object[-1|0_1]2/1(In1)
  Occlusion_Ratio_Object[-1|0_1]2/1(Out1) -> 3D_Sensor_Measurement_3/6  "Occlusion_Ratio_Object[-1|0_1]"
  GetSensorData_3DSensor_3/12(Flag_NearestPnt_Occluded[-1|0|1]) -> Flag_NearestPnt_Occluded[-1|0|1]2/1(In1)
  Flag_NearestPnt_Occluded[-1|0|1]2/1(Out1) -> 3D_Sensor_Measurement_3/7  "Flag_NearestPnt_Occluded[-1|0|1]"

== system ASM_Traffic_V2X_Complete_Model_2/MDLUserInterface/Environment/MDL_DISP/Traffic/TrafficState[] ==
  In1 : Inport
  Out1 : Outport
  wires:
  In1/1 -> Out1/1

== system ASM_Traffic_V2X_Complete_Model_2/MDLUserInterface/Environment/MDL_DISP/Traffic/Traffic_Sign_Sensor ==
  TrafficBus : Inport
  Angle_CoorSys_E[x;y;z][deg] : Subsystem
      mask Display: disp('')
  Angle_Hor_Rel[deg] : Subsystem
      mask Display: disp('')
  Angle_Ver_Rel[] : Subsystem
      mask Display: disp('')
  Bus Selector1 : BusSelector  OutputSignals=Sensors.TrafficSign_Sensor_Dyn.Sensor_Front_1
  Bus Selector2 : BusSelector  OutputSignals=Info.TrafficSignSensor_Dyn_Sfcn_State[],Info.TrafficSignSensor_Dyn_Data_Valid[0|1]
  Distance[m] : Subsystem
      mask Display: disp('')
  GetTrfSgnDataByIndex_1 : Subsystem
  Object_State[] : Subsystem
      mask Display: disp('')
  Object_Stream_ID[] : Subsystem
      mask Display: disp('')
  Parent_Object_ID[] : Subsystem
      mask Display: disp('')
  Pos_CoorSys_E[x;y;z][m] : Subsystem
      mask Display: disp('')
  Pos_CoorSys_S[x;y;z][m] : Subsystem
      mask Display: disp('')
  Select_TrafficSign_1 : Constant
  Sign_Valid[0|1] : Subsystem
      mask Display: disp('')
  TrafficObject_ID[] : Subsystem
      mask Display: disp('')
  TrafficObject_Type[] : Subsystem
      mask Display: disp('')
  TrafficSignSensor_Data_Valid[0|1] : Subsystem
      mask Display: disp('')
  TrafficSignSensor_Sfcn_State[] : Subsystem
      mask Display: disp('')
  TrafficSign_Sensor_Dynamic_ObjectData : Scope  NumInputPorts=4
  TrafficSign_Sensor_Dynamic_ObjectPosition : Scope  NumInputPorts=6
  TrafficSign_Sensor_Dynamic_ObjectPosition1 : Scope  NumInputPorts=8
  TrafficSign_Sensor_Info : Scope  NumInputPorts=2
  Traffic_Sign_Country[] : Subsystem
      mask Display: disp('')
  Traffic_Sign_Lanes[] : Subsystem
      mask Display: disp('')
  Traffic_Sign_Subtype[] : Subsystem
      mask Display: disp('')
  Traffic_Sign_Type[] : Subsystem
      mask Display: disp('')
  Traffic_Sign_Value[] : Subsystem
      mask Display: disp('')
  Traffic_Sign_Visibility[0_100] : Subsystem
      mask Display: disp('')
  wires:
  Bus Selector1/1 -> Bus Selector2/1  "<Sensor_Front_1>"
  TrafficBus/1 -> GetTrfSgnDataByIndex_1/2(TrafficBus), Bus Selector1/1
  Bus Selector2/1 -> TrafficSignSensor_Sfcn_State[]/1(In1)  "<TrafficSignSensor_Dyn_Sfcn_State[]>"
  Bus Selector2/2 -> TrafficSignSensor_Data_Valid[0|1]/1(In1)  "<TrafficSignSensor_Dyn_Data_Valid[0|1]>"
  TrafficSignSensor_Data_Valid[0|1]/1(Out1) -> TrafficSign_Sensor_Info/2  "TrafficSignSensor_Data_Valid[0|1]"
  TrafficSignSensor_Sfcn_State[]/1(Out1) -> TrafficSign_Sensor_Info/1  "TrafficSignSensor_Sfcn_State[]"
  Traffic_Sign_Value[]/1(Out1) -> TrafficSign_Sensor_Dynamic_ObjectPosition1/3  "Traffic_Sign_Value[]"
  Traffic_Sign_Visibility[0_100]/1(Out1) -> TrafficSign_Sensor_Dynamic_ObjectPosition1/5  "Traffic_Sign_Visibility[0_100]"
  Select_TrafficSign_1/1 -> GetTrfSgnDataByIndex_1/1(SelectSignDataByIndex)
  GetTrfSgnDataByIndex_1/1(Traffic_Sign_Valid[0|1]) -> Sign_Valid[0|1]/1(In1)
  GetTrfSgnDataByIndex_1/2(TrafficObject_ID[]) -> TrafficObject_ID[]/1(In1)
  GetTrfSgnDataByIndex_1/3(TrafficObject_Type[]) -> TrafficObject_Type[]/1(In1)
  GetTrfSgnDataByIndex_1/4(Parent_Object_ID[]) -> Parent_Object_ID[]/1(In1)
  TrafficObject_ID[]/1(Out1) -> TrafficSign_Sensor_Dynamic_ObjectData/2  "TrafficObject_ID[]"
  Sign_Valid[0|1]/1(Out1) -> TrafficSign_Sensor_Dynamic_ObjectData/1  "Sign_Valid[0|1]"
  TrafficObject_Type[]/1(Out1) -> TrafficSign_Sensor_Dynamic_ObjectData/3  "TrafficObject_Type[]"
  Parent_Object_ID[]/1(Out1) -> TrafficSign_Sensor_Dynamic_ObjectData/4  "Parent_Object_ID[]"
  GetTrfSgnDataByIndex_1/5(Pos_CoorSys_E[x;y;z][m]) -> Pos_CoorSys_E[x;y;z][m]/1(In1)
  GetTrfSgnDataByIndex_1/6(Angle_CoorSys_E[x;y;z][deg]) -> Angle_CoorSys_E[x;y;z][deg]/1(In1)
  GetTrfSgnDataByIndex_1/7(Pos_CoorSys_S[x;y;z][m]) -> Pos_CoorSys_S[x;y;z][m]/1(In1)
  GetTrfSgnDataByIndex_1/8(Angle_Hor_Rel[deg]) -> Angle_Hor_Rel[deg]/1(In1)
  GetTrfSgnDataByIndex_1/9(Angle_Ver_Rel[deg]) -> Angle_Ver_Rel[]/1(In1)
  GetTrfSgnDataByIndex_1/10(Distance[m]) -> Distance[m]/1(In1)
  Pos_CoorSys_E[x;y;z][m]/1(Out1) -> TrafficSign_Sensor_Dynamic_ObjectPosition/1  "Pos_CoorSys_E[x;y;z][m]"
  Angle_CoorSys_E[x;y;z][deg]/1(Out1) -> TrafficSign_Sensor_Dynamic_ObjectPosition/2  "Angle_CoorSys_E[x;y;z][deg]"
  Pos_CoorSys_S[x;y;z][m]/1(Out1) -> TrafficSign_Sensor_Dynamic_ObjectPosition/3  "Pos_CoorSys_S[x;y;z][m]"
  Angle_Hor_Rel[deg]/1(Out1) -> TrafficSign_Sensor_Dynamic_ObjectPosition/4  "Angle_Hor_Rel[deg]"
  Angle_Ver_Rel[]/1(Out1) -> TrafficSign_Sensor_Dynamic_ObjectPosition/5  "Angle_Ver_Rel[]"
  Distance[m]/1(Out1) -> TrafficSign_Sensor_Dynamic_ObjectPosition/6  "Distance[m]"
  GetTrfSgnDataByIndex_1/11(Traffic_Sign_Type[]) -> Traffic_Sign_Type[]/1(In1)
  GetTrfSgnDataByIndex_1/12(Traffic_Sign_Subtype[]) -> Traffic_Sign_Subtype[]/1(In1)
  GetTrfSgnDataByIndex_1/13(Traffic_Sign_Value[]) -> Traffic_Sign_Value[]/1(In1)
  GetTrfSgnDataByIndex_1/14(Traffic_Sign_Country[]) -> Traffic_Sign_Country[]/1(In1)
  Traffic_Sign_Type[]/1(Out1) -> TrafficSign_Sensor_Dynamic_ObjectPosition1/1  "Traffic_Sign_Type[]"
  Traffic_Sign_Subtype[]/1(Out1) -> TrafficSign_Sensor_Dynamic_ObjectPosition1/2  "Traffic_Sign_Subtype[]"
  GetTrfSgnDataByIndex_1/15(Traffic_Sign_Visibility[0_100]) -> Traffic_Sign_Visibility[0_100]/1(In1)
  Traffic_Sign_Country[]/1(Out1) -> TrafficSign_Sensor_Dynamic_ObjectPosition1/4  "Traffic_Sign_Country[]"
  GetTrfSgnDataByIndex_1/16(Object_State[]) -> Object_State[]/1(In1)
  GetTrfSgnDataByIndex_1/17(Object_Stream_ID[]) -> Object_Stream_ID[]/1(In1)
  GetTrfSgnDataByIndex_1/18(Traffic_Sign_Lanes[]) -> Traffic_Sign_Lanes[]/1(In1)
  Object_State[]/1(Out1) -> TrafficSign_Sensor_Dynamic_ObjectPosition1/6  "Object_State[]"
  Object_Stream_ID[]/1(Out1) -> TrafficSign_Sensor_Dynamic_ObjectPosition1/7  "Object_Stream_ID[]"
  Traffic_Sign_Lanes[]/1(Out1) -> TrafficSign_Sensor_Dynamic_ObjectPosition1/8  "Traffic_Sign_Lanes[]"

== system ASM_Traffic_V2X_Complete_Model_2/MDLUserInterface/Environment/MDL_PAR/Fellow_VehicleLights/Fellow10_VehicleLights ==
  Bus Creator1 : BusCreator  Inputs=3
  SW_BrakeLight[0Off|1On] : Constant  Value=0
  SW_ManualControl_Lights[1Scheduler|2Manual] : Constant
  SW_TurnLights[0Off|1Left|2Right|3Both] : Constant  Value=0
  Out1 : Outport
  wires:
  Bus Creator1/1 -> Out1/1
  SW_BrakeLight[0Off|1On]/1 -> Bus Creator1/2  "SW_BrakeLight[0Off|1On]"
  SW_TurnLights[0Off|1Left|2Right|3Both]/1 -> Bus Creator1/3  "SW_TurnLights[0Off|1Left|2Right|3Both]"
  SW_ManualControl_Lights[1Scheduler|2Manual]/1 -> Bus Creator1/1  "SW_ManualControl_Lights[1Scheduler|2Manual]"

== system ASM_Traffic_V2X_Complete_Model_2/MDLUserInterface/Environment/MDL_PAR/Fellow_VehicleLights/Fellow11_VehicleLights ==
  Bus Creator1 : BusCreator  Inputs=3
  SW_BrakeLight[0Off|1On] : Constant  Value=0
  SW_ManualControl_Lights[1Scheduler|2Manual] : Constant
  SW_TurnLights[0Off|1Left|2Right|3Both] : Constant  Value=0
  Out1 : Outport
  wires:
  SW_ManualControl_Lights[1Scheduler|2Manual]/1 -> Bus Creator1/1  "SW_ManualControl_Lights[1Scheduler|2Manual]"
  SW_TurnLights[0Off|1Left|2Right|3Both]/1 -> Bus Creator1/3  "SW_TurnLights[0Off|1Left|2Right|3Both]"
  SW_BrakeLight[0Off|1On]/1 -> Bus Creator1/2  "SW_BrakeLight[0Off|1On]"
  Bus Creator1/1 -> Out1/1

== system ASM_Traffic_V2X_Complete_Model_2/MDLUserInterface/Environment/MDL_PAR/Fellow_VehicleLights/Fellow12_VehicleLights ==
  Bus Creator1 : BusCreator  Inputs=3
  SW_BrakeLight[0Off|1On] : Constant  Value=0
  SW_ManualControl_Lights[1Scheduler|2Manual] : Constant
  SW_TurnLights[0Off|1Left|2Right|3Both] : Constant  Value=0
  Out1 : Outport
  wires:
  Bus Creator1/1 -> Out1/1
  SW_BrakeLight[0Off|1On]/1 -> Bus Creator1/2  "SW_BrakeLight[0Off|1On]"
  SW_TurnLights[0Off|1Left|2Right|3Both]/1 -> Bus Creator1/3  "SW_TurnLights[0Off|1Left|2Right|3Both]"
  SW_ManualControl_Lights[1Scheduler|2Manual]/1 -> Bus Creator1/1  "SW_ManualControl_Lights[1Scheduler|2Manual]"
